simulink model "Const1"  (Simulink 7.9)
settings: Solver=ode45  StartTime=0.0  StopTime=10.0  RelTol=1e-3
settings Model: Creator=boakes  LastModifiedBy=boakes

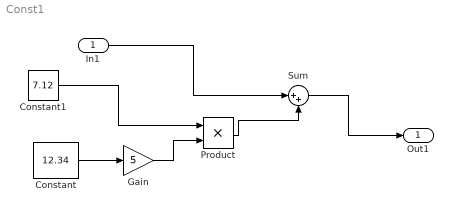
== system Const1 ==
  In1 : Inport
  Constant : Constant  Value=12.34
  Constant1 : Constant  Value=7.12
  Gain : Gain  Gain=5
  Product : Product  RndMeth=Zero
  Sum : Sum  Inputs=|++
  Out1 : Outport
  wires:
  Constant1/1 -> Product/1
  In1/1 -> Sum/1
  Product/1 -> Sum/2
  Constant/1 -> Gain/1
  Gain/1 -> Product/2
  Sum/1 -> Out1/1
